simulink model "Charge_2_V1"  (R2017b)
settings: Solver=FixedStepDiscrete  StartTime=0.0  StopTime=1  FixedStep=0.001  RelTol=1e-3
PreLoadFcn:
  | librarySetup
  | eval([bdroot,'_startup']) %Calling [modelName]_startup.m
undefined symbols (not defined in the file or in its folder): A0, A1, Car1__Authorize, Car2_Authorize, CON2, CON3, CON4, Control_Mode_In, CurrentSP, D10, D12, D13, D2, D3, D4, D5, D6, D7, D8, Frequency_High_Point, Frequency_Low_Point, Frequency_Mid_high, Frequency_Mid_low, HVol_High_Point, HVol_Low_Point, HVol_Mid_high, HVol_Mid_low, HVoltage_Factor, SeconCar_ThreePhase, V_Current_five, V_Current_four, V_Current_one, V_Current_six, V_Current_three, V_Current_two, V_Frequency, V_MaxPliot, V_MinPliot, Vol_High_Point, Vol_Low_Point, Vol_Mid_high, Vol_Mid_low, Voltage_Factor, Voltage_Mode_Test
libraries: simulink x331, HANcoder_STM32_Target x30, powerlib_meascontrol x8, simulink_extras x2
(part 5 of 13)

== system Charge_2_V1/HANcoder STM32 Target - E407-STM32 algorithm/Energy Meter1/Energy_Meter_Recieve/Current_Meter/Read_Gyro13 ==
  Trigger : TriggerPort  VariantControl=Variant
  UART receive : Subsystem  AncestorBlock=HANcoder_STM32_Target/STM32-E407/UART/UART receive  mask(UART receive){channel=UART2: Con. PD-8 & Con. PD-9 (PD5 & PD6), useStatusOut=off, tsamp=-1}
      mask prompts: useStatusOut "Use status outport"; tsamp "Sample time"
      mask help:
      | Function
      | ==========
      | Reads a byte from the UART reception buffer.
      |
      | Parameters per channel
      | ======================
      | - Select channel
      | - Select if the status output should be enabled.
      |
      | Outputs
      | =======
      | - The value of the receive byte.
      | - When the status output is 0, the reception buffer was empty.
      mask init:
      | uartChannelInfoStr = sfcn_uart_receive_mcb(2, channel, useStatusOut);
      settings: MoveFcn=drawLogos
      mask Help: web('sfcn_uart_receive.html')
      mask TypeOptions channel: UART1: Con. 3-D1 & Con. 3-D0 (PB6 & PB7) | UART2: Con. PD-8 & Con. PD-9 (PD5 & PD6) | UART3: Con. PD-11 & Con. PD-12 (PD8 & PD9) | UART6: Con. UEXT-3 & Con. UEXT-4 (PC6 & PC7)
      mask Display: fprintf('UART receive\n%s', uartChannelInfoStr);patch([240 246 246],[8 14 2],[1 0 0]);patch([248 248 254],[14 2 8],[0 0 0.35]);
  Out1 : Outport
  wires:
  UART receive/1(Out1) -> Out1/1

== system Charge_2_V1/HANcoder STM32 Target - E407-STM32 algorithm/Energy Meter1/Energy_Meter_Recieve/Current_Meter/Read_Gyro14 ==
  Trigger : TriggerPort  VariantControl=Variant
  UART receive : Subsystem  AncestorBlock=HANcoder_STM32_Target/STM32-E407/UART/UART receive  mask(UART receive){channel=UART2: Con. PD-8 & Con. PD-9 (PD5 & PD6), useStatusOut=off, tsamp=-1}
      mask prompts: useStatusOut "Use status outport"; tsamp "Sample time"
      mask help:
      | Function
      | ==========
      | Reads a byte from the UART reception buffer.
      |
      | Parameters per channel
      | ======================
      | - Select channel
      | - Select if the status output should be enabled.
      |
      | Outputs
      | =======
      | - The value of the receive byte.
      | - When the status output is 0, the reception buffer was empty.
      mask init:
      | uartChannelInfoStr = sfcn_uart_receive_mcb(2, channel, useStatusOut);
      settings: MoveFcn=drawLogos
      mask Help: web('sfcn_uart_receive.html')
      mask TypeOptions channel: UART1: Con. 3-D1 & Con. 3-D0 (PB6 & PB7) | UART2: Con. PD-8 & Con. PD-9 (PD5 & PD6) | UART3: Con. PD-11 & Con. PD-12 (PD8 & PD9) | UART6: Con. UEXT-3 & Con. UEXT-4 (PC6 & PC7)
      mask Display: fprintf('UART receive\n%s', uartChannelInfoStr);patch([240 246 246],[8 14 2],[1 0 0]);patch([248 248 254],[14 2 8],[0 0 0.35]);
  Out1 : Outport
  wires:
  UART receive/1(Out1) -> Out1/1

== system Charge_2_V1/HANcoder STM32 Target - E407-STM32 algorithm/Energy Meter1/Energy_Meter_Recieve/Current_Meter/Read_Gyro15 ==
  Trigger : TriggerPort  VariantControl=Variant
  UART receive : Subsystem  AncestorBlock=HANcoder_STM32_Target/STM32-E407/UART/UART receive  mask(UART receive){channel=UART2: Con. PD-8 & Con. PD-9 (PD5 & PD6), useStatusOut=off, tsamp=-1}
      mask prompts: useStatusOut "Use status outport"; tsamp "Sample time"
      mask help:
      | Function
      | ==========
      | Reads a byte from the UART reception buffer.
      |
      | Parameters per channel
      | ======================
      | - Select channel
      | - Select if the status output should be enabled.
      |
      | Outputs
      | =======
      | - The value of the receive byte.
      | - When the status output is 0, the reception buffer was empty.
      mask init:
      | uartChannelInfoStr = sfcn_uart_receive_mcb(2, channel, useStatusOut);
      settings: MoveFcn=drawLogos
      mask Help: web('sfcn_uart_receive.html')
      mask TypeOptions channel: UART1: Con. 3-D1 & Con. 3-D0 (PB6 & PB7) | UART2: Con. PD-8 & Con. PD-9 (PD5 & PD6) | UART3: Con. PD-11 & Con. PD-12 (PD8 & PD9) | UART6: Con. UEXT-3 & Con. UEXT-4 (PC6 & PC7)
      mask Display: fprintf('UART receive\n%s', uartChannelInfoStr);patch([240 246 246],[8 14 2],[1 0 0]);patch([248 248 254],[14 2 8],[0 0 0.35]);
  Out1 : Outport
  wires:
  UART receive/1(Out1) -> Out1/1

== system Charge_2_V1/HANcoder STM32 Target - E407-STM32 algorithm/Energy Meter1/Energy_Meter_Recieve/Current_Meter/Read_Gyro16 ==
  Trigger : TriggerPort  VariantControl=Variant
  UART receive : Subsystem  AncestorBlock=HANcoder_STM32_Target/STM32-E407/UART/UART receive  mask(UART receive){channel=UART2: Con. PD-8 & Con. PD-9 (PD5 & PD6), useStatusOut=off, tsamp=-1}
      mask prompts: useStatusOut "Use status outport"; tsamp "Sample time"
      mask help:
      | Function
      | ==========
      | Reads a byte from the UART reception buffer.
      |
      | Parameters per channel
      | ======================
      | - Select channel
      | - Select if the status output should be enabled.
      |
      | Outputs
      | =======
      | - The value of the receive byte.
      | - When the status output is 0, the reception buffer was empty.
      mask init:
      | uartChannelInfoStr = sfcn_uart_receive_mcb(2, channel, useStatusOut);
      settings: MoveFcn=drawLogos
      mask Help: web('sfcn_uart_receive.html')
      mask TypeOptions channel: UART1: Con. 3-D1 & Con. 3-D0 (PB6 & PB7) | UART2: Con. PD-8 & Con. PD-9 (PD5 & PD6) | UART3: Con. PD-11 & Con. PD-12 (PD8 & PD9) | UART6: Con. UEXT-3 & Con. UEXT-4 (PC6 & PC7)
      mask Display: fprintf('UART receive\n%s', uartChannelInfoStr);patch([240 246 246],[8 14 2],[1 0 0]);patch([248 248 254],[14 2 8],[0 0 0.35]);
  Out1 : Outport
  wires:
  UART receive/1(Out1) -> Out1/1

== system Charge_2_V1/HANcoder STM32 Target - E407-STM32 algorithm/Energy Meter1/Energy_Meter_Recieve/Current_Meter/Read_Gyro17 ==
  Trigger : TriggerPort  VariantControl=Variant
  UART receive : Subsystem  AncestorBlock=HANcoder_STM32_Target/STM32-E407/UART/UART receive  mask(UART receive){channel=UART2: Con. PD-8 & Con. PD-9 (PD5 & PD6), useStatusOut=off, tsamp=-1}
      mask prompts: useStatusOut "Use status outport"; tsamp "Sample time"
      mask help:
      | Function
      | ==========
      | Reads a byte from the UART reception buffer.
      |
      | Parameters per channel
      | ======================
      | - Select channel
      | - Select if the status output should be enabled.
      |
      | Outputs
      | =======
      | - The value of the receive byte.
      | - When the status output is 0, the reception buffer was empty.
      mask init:
      | uartChannelInfoStr = sfcn_uart_receive_mcb(2, channel, useStatusOut);
      settings: MoveFcn=drawLogos
      mask Help: web('sfcn_uart_receive.html')
      mask TypeOptions channel: UART1: Con. 3-D1 & Con. 3-D0 (PB6 & PB7) | UART2: Con. PD-8 & Con. PD-9 (PD5 & PD6) | UART3: Con. PD-11 & Con. PD-12 (PD8 & PD9) | UART6: Con. UEXT-3 & Con. UEXT-4 (PC6 & PC7)
      mask Display: fprintf('UART receive\n%s', uartChannelInfoStr);patch([240 246 246],[8 14 2],[1 0 0]);patch([248 248 254],[14 2 8],[0 0 0.35]);
  Out1 : Outport
  wires:
  UART receive/1(Out1) -> Out1/1

== system Charge_2_V1/HANcoder STM32 Target - E407-STM32 algorithm/Energy Meter1/Energy_Meter_Recieve/Current_Meter/Read_Gyro18 ==
  Trigger : TriggerPort  VariantControl=Variant
  UART receive : Subsystem  AncestorBlock=HANcoder_STM32_Target/STM32-E407/UART/UART receive  mask(UART receive){channel=UART2: Con. PD-8 & Con. PD-9 (PD5 & PD6), useStatusOut=off, tsamp=-1}
      mask prompts: useStatusOut "Use status outport"; tsamp "Sample time"
      mask help:
      | Function
      | ==========
      | Reads a byte from the UART reception buffer.
      |
      | Parameters per channel
      | ======================
      | - Select channel
      | - Select if the status output should be enabled.
      |
      | Outputs
      | =======
      | - The value of the receive byte.
      | - When the status output is 0, the reception buffer was empty.
      mask init:
      | uartChannelInfoStr = sfcn_uart_receive_mcb(2, channel, useStatusOut);
      settings: MoveFcn=drawLogos
      mask Help: web('sfcn_uart_receive.html')
      mask TypeOptions channel: UART1: Con. 3-D1 & Con. 3-D0 (PB6 & PB7) | UART2: Con. PD-8 & Con. PD-9 (PD5 & PD6) | UART3: Con. PD-11 & Con. PD-12 (PD8 & PD9) | UART6: Con. UEXT-3 & Con. UEXT-4 (PC6 & PC7)
      mask Display: fprintf('UART receive\n%s', uartChannelInfoStr);patch([240 246 246],[8 14 2],[1 0 0]);patch([248 248 254],[14 2 8],[0 0 0.35]);
  Out1 : Outport
  wires:
  UART receive/1(Out1) -> Out1/1

== system Charge_2_V1/HANcoder STM32 Target - E407-STM32 algorithm/Energy Meter1/Energy_Meter_Recieve/Current_Meter/Read_Gyro2 ==
  Trigger : TriggerPort  VariantControl=Variant
  UART receive : Subsystem  AncestorBlock=HANcoder_STM32_Target/STM32-E407/UART/UART receive  mask(UART receive){channel=UART2: Con. PD-8 & Con. PD-9 (PD5 & PD6), useStatusOut=off, tsamp=-1}
      mask prompts: useStatusOut "Use status outport"; tsamp "Sample time"
      mask help:
      | Function
      | ==========
      | Reads a byte from the UART reception buffer.
      |
      | Parameters per channel
      | ======================
      | - Select channel
      | - Select if the status output should be enabled.
      |
      | Outputs
      | =======
      | - The value of the receive byte.
      | - When the status output is 0, the reception buffer was empty.
      mask init:
      | uartChannelInfoStr = sfcn_uart_receive_mcb(2, channel, useStatusOut);
      settings: MoveFcn=drawLogos
      mask Help: web('sfcn_uart_receive.html')
      mask TypeOptions channel: UART1: Con. 3-D1 & Con. 3-D0 (PB6 & PB7) | UART2: Con. PD-8 & Con. PD-9 (PD5 & PD6) | UART3: Con. PD-11 & Con. PD-12 (PD8 & PD9) | UART6: Con. UEXT-3 & Con. UEXT-4 (PC6 & PC7)
      mask Display: fprintf('UART receive\n%s', uartChannelInfoStr);patch([240 246 246],[8 14 2],[1 0 0]);patch([248 248 254],[14 2 8],[0 0 0.35]);
  Out1 : Outport
  wires:
  UART receive/1(Out1) -> Out1/1

== system Charge_2_V1/HANcoder STM32 Target - E407-STM32 algorithm/Energy Meter1/Energy_Meter_Recieve/Current_Meter/Read_Gyro3 ==
  Trigger : TriggerPort  VariantControl=Variant
  UART receive : Subsystem  AncestorBlock=HANcoder_STM32_Target/STM32-E407/UART/UART receive  mask(UART receive){channel=UART2: Con. PD-8 & Con. PD-9 (PD5 & PD6), useStatusOut=off, tsamp=-1}
      mask prompts: useStatusOut "Use status outport"; tsamp "Sample time"
      mask help:
      | Function
      | ==========
      | Reads a byte from the UART reception buffer.
      |
      | Parameters per channel
      | ======================
      | - Select channel
      | - Select if the status output should be enabled.
      |
      | Outputs
      | =======
      | - The value of the receive byte.
      | - When the status output is 0, the reception buffer was empty.
      mask init:
      | uartChannelInfoStr = sfcn_uart_receive_mcb(2, channel, useStatusOut);
      settings: MoveFcn=drawLogos
      mask Help: web('sfcn_uart_receive.html')
      mask TypeOptions channel: UART1: Con. 3-D1 & Con. 3-D0 (PB6 & PB7) | UART2: Con. PD-8 & Con. PD-9 (PD5 & PD6) | UART3: Con. PD-11 & Con. PD-12 (PD8 & PD9) | UART6: Con. UEXT-3 & Con. UEXT-4 (PC6 & PC7)
      mask Display: fprintf('UART receive\n%s', uartChannelInfoStr);patch([240 246 246],[8 14 2],[1 0 0]);patch([248 248 254],[14 2 8],[0 0 0.35]);
  Out1 : Outport
  wires:
  UART receive/1(Out1) -> Out1/1

== system Charge_2_V1/HANcoder STM32 Target - E407-STM32 algorithm/Energy Meter1/Energy_Meter_Recieve/Current_Meter/Read_Gyro4 ==
  Trigger : TriggerPort  VariantControl=Variant
  UART receive : Subsystem  AncestorBlock=HANcoder_STM32_Target/STM32-E407/UART/UART receive  mask(UART receive){channel=UART2: Con. PD-8 & Con. PD-9 (PD5 & PD6), useStatusOut=off, tsamp=-1}
      mask prompts: useStatusOut "Use status outport"; tsamp "Sample time"
      mask help:
      | Function
      | ==========
      | Reads a byte from the UART reception buffer.
      |
      | Parameters per channel
      | ======================
      | - Select channel
      | - Select if the status output should be enabled.
      |
      | Outputs
      | =======
      | - The value of the receive byte.
      | - When the status output is 0, the reception buffer was empty.
      mask init:
      | uartChannelInfoStr = sfcn_uart_receive_mcb(2, channel, useStatusOut);
      settings: MoveFcn=drawLogos
      mask Help: web('sfcn_uart_receive.html')
      mask TypeOptions channel: UART1: Con. 3-D1 & Con. 3-D0 (PB6 & PB7) | UART2: Con. PD-8 & Con. PD-9 (PD5 & PD6) | UART3: Con. PD-11 & Con. PD-12 (PD8 & PD9) | UART6: Con. UEXT-3 & Con. UEXT-4 (PC6 & PC7)
      mask Display: fprintf('UART receive\n%s', uartChannelInfoStr);patch([240 246 246],[8 14 2],[1 0 0]);patch([248 248 254],[14 2 8],[0 0 0.35]);
  Out1 : Outport
  wires:
  UART receive/1(Out1) -> Out1/1

== system Charge_2_V1/HANcoder STM32 Target - E407-STM32 algorithm/Energy Meter1/Energy_Meter_Recieve/Current_Meter/Read_Gyro5 ==
  Trigger : TriggerPort  VariantControl=Variant
  UART receive : Subsystem  AncestorBlock=HANcoder_STM32_Target/STM32-E407/UART/UART receive  mask(UART receive){channel=UART2: Con. PD-8 & Con. PD-9 (PD5 & PD6), useStatusOut=off, tsamp=-1}
      mask prompts: useStatusOut "Use status outport"; tsamp "Sample time"
      mask help:
      | Function
      | ==========
      | Reads a byte from the UART reception buffer.
      |
      | Parameters per channel
      | ======================
      | - Select channel
      | - Select if the status output should be enabled.
      |
      | Outputs
      | =======
      | - The value of the receive byte.
      | - When the status output is 0, the reception buffer was empty.
      mask init:
      | uartChannelInfoStr = sfcn_uart_receive_mcb(2, channel, useStatusOut);
      settings: MoveFcn=drawLogos
      mask Help: web('sfcn_uart_receive.html')
      mask TypeOptions channel: UART1: Con. 3-D1 & Con. 3-D0 (PB6 & PB7) | UART2: Con. PD-8 & Con. PD-9 (PD5 & PD6) | UART3: Con. PD-11 & Con. PD-12 (PD8 & PD9) | UART6: Con. UEXT-3 & Con. UEXT-4 (PC6 & PC7)
      mask Display: fprintf('UART receive\n%s', uartChannelInfoStr);patch([240 246 246],[8 14 2],[1 0 0]);patch([248 248 254],[14 2 8],[0 0 0.35]);
  Out1 : Outport
  wires:
  UART receive/1(Out1) -> Out1/1

== system Charge_2_V1/HANcoder STM32 Target - E407-STM32 algorithm/Energy Meter1/Energy_Meter_Recieve/Current_Meter/Read_Gyro6 ==
  Trigger : TriggerPort  VariantControl=Variant
  UART receive : Subsystem  AncestorBlock=HANcoder_STM32_Target/STM32-E407/UART/UART receive  mask(UART receive){channel=UART2: Con. PD-8 & Con. PD-9 (PD5 & PD6), useStatusOut=off, tsamp=-1}
      mask prompts: useStatusOut "Use status outport"; tsamp "Sample time"
      mask help:
      | Function
      | ==========
      | Reads a byte from the UART reception buffer.
      |
      | Parameters per channel
      | ======================
      | - Select channel
      | - Select if the status output should be enabled.
      |
      | Outputs
      | =======
      | - The value of the receive byte.
      | - When the status output is 0, the reception buffer was empty.
      mask init:
      | uartChannelInfoStr = sfcn_uart_receive_mcb(2, channel, useStatusOut);
      settings: MoveFcn=drawLogos
      mask Help: web('sfcn_uart_receive.html')
      mask TypeOptions channel: UART1: Con. 3-D1 & Con. 3-D0 (PB6 & PB7) | UART2: Con. PD-8 & Con. PD-9 (PD5 & PD6) | UART3: Con. PD-11 & Con. PD-12 (PD8 & PD9) | UART6: Con. UEXT-3 & Con. UEXT-4 (PC6 & PC7)
      mask Display: fprintf('UART receive\n%s', uartChannelInfoStr);patch([240 246 246],[8 14 2],[1 0 0]);patch([248 248 254],[14 2 8],[0 0 0.35]);
  Out1 : Outport
  wires:
  UART receive/1(Out1) -> Out1/1

== system Charge_2_V1/HANcoder STM32 Target - E407-STM32 algorithm/Energy Meter1/Energy_Meter_Recieve/Current_Meter/Read_Gyro7 ==
  Trigger : TriggerPort  VariantControl=Variant
  UART receive : Subsystem  AncestorBlock=HANcoder_STM32_Target/STM32-E407/UART/UART receive  mask(UART receive){channel=UART2: Con. PD-8 & Con. PD-9 (PD5 & PD6), useStatusOut=off, tsamp=-1}
      mask prompts: useStatusOut "Use status outport"; tsamp "Sample time"
      mask help:
      | Function
      | ==========
      | Reads a byte from the UART reception buffer.
      |
      | Parameters per channel
      | ======================
      | - Select channel
      | - Select if the status output should be enabled.
      |
      | Outputs
      | =======
      | - The value of the receive byte.
      | - When the status output is 0, the reception buffer was empty.
      mask init:
      | uartChannelInfoStr = sfcn_uart_receive_mcb(2, channel, useStatusOut);
      settings: MoveFcn=drawLogos
      mask Help: web('sfcn_uart_receive.html')
      mask TypeOptions channel: UART1: Con. 3-D1 & Con. 3-D0 (PB6 & PB7) | UART2: Con. PD-8 & Con. PD-9 (PD5 & PD6) | UART3: Con. PD-11 & Con. PD-12 (PD8 & PD9) | UART6: Con. UEXT-3 & Con. UEXT-4 (PC6 & PC7)
      mask Display: fprintf('UART receive\n%s', uartChannelInfoStr);patch([240 246 246],[8 14 2],[1 0 0]);patch([248 248 254],[14 2 8],[0 0 0.35]);
  Out1 : Outport
  wires:
  UART receive/1(Out1) -> Out1/1

== system Charge_2_V1/HANcoder STM32 Target - E407-STM32 algorithm/Energy Meter1/Energy_Meter_Recieve/Current_Meter/Read_Gyro8 ==
  Trigger : TriggerPort  VariantControl=Variant
  UART receive : Subsystem  AncestorBlock=HANcoder_STM32_Target/STM32-E407/UART/UART receive  mask(UART receive){channel=UART2: Con. PD-8 & Con. PD-9 (PD5 & PD6), useStatusOut=off, tsamp=-1}
      mask prompts: useStatusOut "Use status outport"; tsamp "Sample time"
      mask help:
      | Function
      | ==========
      | Reads a byte from the UART reception buffer.
      |
      | Parameters per channel
      | ======================
      | - Select channel
      | - Select if the status output should be enabled.
      |
      | Outputs
      | =======
      | - The value of the receive byte.
      | - When the status output is 0, the reception buffer was empty.
      mask init:
      | uartChannelInfoStr = sfcn_uart_receive_mcb(2, channel, useStatusOut);
      settings: MoveFcn=drawLogos
      mask Help: web('sfcn_uart_receive.html')
      mask TypeOptions channel: UART1: Con. 3-D1 & Con. 3-D0 (PB6 & PB7) | UART2: Con. PD-8 & Con. PD-9 (PD5 & PD6) | UART3: Con. PD-11 & Con. PD-12 (PD8 & PD9) | UART6: Con. UEXT-3 & Con. UEXT-4 (PC6 & PC7)
      mask Display: fprintf('UART receive\n%s', uartChannelInfoStr);patch([240 246 246],[8 14 2],[1 0 0]);patch([248 248 254],[14 2 8],[0 0 0.35]);
  Out1 : Outport
  wires:
  UART receive/1(Out1) -> Out1/1

== system Charge_2_V1/HANcoder STM32 Target - E407-STM32 algorithm/Energy Meter1/Energy_Meter_Recieve/Current_Meter/Read_Gyro9 ==
  Trigger : TriggerPort  VariantControl=Variant
  UART receive : Subsystem  AncestorBlock=HANcoder_STM32_Target/STM32-E407/UART/UART receive  mask(UART receive){channel=UART2: Con. PD-8 & Con. PD-9 (PD5 & PD6), useStatusOut=off, tsamp=-1}
      mask prompts: useStatusOut "Use status outport"; tsamp "Sample time"
      mask help:
      | Function
      | ==========
      | Reads a byte from the UART reception buffer.
      |
      | Parameters per channel
      | ======================
      | - Select channel
      | - Select if the status output should be enabled.
      |
      | Outputs
      | =======
      | - The value of the receive byte.
      | - When the status output is 0, the reception buffer was empty.
      mask init:
      | uartChannelInfoStr = sfcn_uart_receive_mcb(2, channel, useStatusOut);
      settings: MoveFcn=drawLogos
      mask Help: web('sfcn_uart_receive.html')
      mask TypeOptions channel: UART1: Con. 3-D1 & Con. 3-D0 (PB6 & PB7) | UART2: Con. PD-8 & Con. PD-9 (PD5 & PD6) | UART3: Con. PD-11 & Con. PD-12 (PD8 & PD9) | UART6: Con. UEXT-3 & Con. UEXT-4 (PC6 & PC7)
      mask Display: fprintf('UART receive\n%s', uartChannelInfoStr);patch([240 246 246],[8 14 2],[1 0 0]);patch([248 248 254],[14 2 8],[0 0 0.35]);
  Out1 : Outport
  wires:
  UART receive/1(Out1) -> Out1/1

== system Charge_2_V1/HANcoder STM32 Target - E407-STM32 algorithm/Energy Meter1/Energy_Meter_Recieve/Fequency/Read_Gyro ==
  Trigger : TriggerPort  VariantControl=Variant
  UART receive : Subsystem  AncestorBlock=HANcoder_STM32_Target/STM32-E407/UART/UART receive  mask(UART receive){channel=UART2: Con. PD-8 & Con. PD-9 (PD5 & PD6), useStatusOut=off, tsamp=-1}
      mask prompts: useStatusOut "Use status outport"; tsamp "Sample time"
      mask help:
      | Function
      | ==========
      | Reads a byte from the UART reception buffer.
      |
      | Parameters per channel
      | ======================
      | - Select channel
      | - Select if the status output should be enabled.
      |
      | Outputs
      | =======
      | - The value of the receive byte.
      | - When the status output is 0, the reception buffer was empty.
      mask init:
      | uartChannelInfoStr = sfcn_uart_receive_mcb(2, channel, useStatusOut);
      settings: MoveFcn=drawLogos
      mask Help: web('sfcn_uart_receive.html')
      mask TypeOptions channel: UART1: Con. 3-D1 & Con. 3-D0 (PB6 & PB7) | UART2: Con. PD-8 & Con. PD-9 (PD5 & PD6) | UART3: Con. PD-11 & Con. PD-12 (PD8 & PD9) | UART6: Con. UEXT-3 & Con. UEXT-4 (PC6 & PC7)
      mask Display: fprintf('UART receive\n%s', uartChannelInfoStr);patch([240 246 246],[8 14 2],[1 0 0]);patch([248 248 254],[14 2 8],[0 0 0.35]);
  Out1 : Outport
  wires:
  UART receive/1(Out1) -> Out1/1

== system Charge_2_V1/HANcoder STM32 Target - E407-STM32 algorithm/Energy Meter1/Energy_Meter_Recieve/Fequency/Read_Gyro1 ==
  Trigger : TriggerPort  VariantControl=Variant
  UART receive : Subsystem  AncestorBlock=HANcoder_STM32_Target/STM32-E407/UART/UART receive  mask(UART receive){channel=UART2: Con. PD-8 & Con. PD-9 (PD5 & PD6), useStatusOut=off, tsamp=-1}
      mask prompts: useStatusOut "Use status outport"; tsamp "Sample time"
      mask help:
      | Function
      | ==========
      | Reads a byte from the UART reception buffer.
      |
      | Parameters per channel
      | ======================
      | - Select channel
      | - Select if the status output should be enabled.
      |
      | Outputs
      | =======
      | - The value of the receive byte.
      | - When the status output is 0, the reception buffer was empty.
      mask init:
      | uartChannelInfoStr = sfcn_uart_receive_mcb(2, channel, useStatusOut);
      settings: MoveFcn=drawLogos
      mask Help: web('sfcn_uart_receive.html')
      mask TypeOptions channel: UART1: Con. 3-D1 & Con. 3-D0 (PB6 & PB7) | UART2: Con. PD-8 & Con. PD-9 (PD5 & PD6) | UART3: Con. PD-11 & Con. PD-12 (PD8 & PD9) | UART6: Con. UEXT-3 & Con. UEXT-4 (PC6 & PC7)
      mask Display: fprintf('UART receive\n%s', uartChannelInfoStr);patch([240 246 246],[8 14 2],[1 0 0]);patch([248 248 254],[14 2 8],[0 0 0.35]);
  Out1 : Outport
  wires:
  UART receive/1(Out1) -> Out1/1

== system Charge_2_V1/HANcoder STM32 Target - E407-STM32 algorithm/Energy Meter1/Energy_Meter_Recieve/Fequency/Read_Gyro10 ==
  Trigger : TriggerPort  VariantControl=Variant
  UART receive : Subsystem  AncestorBlock=HANcoder_STM32_Target/STM32-E407/UART/UART receive  mask(UART receive){channel=UART2: Con. PD-8 & Con. PD-9 (PD5 & PD6), useStatusOut=off, tsamp=-1}
      mask prompts: useStatusOut "Use status outport"; tsamp "Sample time"
      mask help:
      | Function
      | ==========
      | Reads a byte from the UART reception buffer.
      |
      | Parameters per channel
      | ======================
      | - Select channel
      | - Select if the status output should be enabled.
      |
      | Outputs
      | =======
      | - The value of the receive byte.
      | - When the status output is 0, the reception buffer was empty.
      mask init:
      | uartChannelInfoStr = sfcn_uart_receive_mcb(2, channel, useStatusOut);
      settings: MoveFcn=drawLogos
      mask Help: web('sfcn_uart_receive.html')
      mask TypeOptions channel: UART1: Con. 3-D1 & Con. 3-D0 (PB6 & PB7) | UART2: Con. PD-8 & Con. PD-9 (PD5 & PD6) | UART3: Con. PD-11 & Con. PD-12 (PD8 & PD9) | UART6: Con. UEXT-3 & Con. UEXT-4 (PC6 & PC7)
      mask Display: fprintf('UART receive\n%s', uartChannelInfoStr);patch([240 246 246],[8 14 2],[1 0 0]);patch([248 248 254],[14 2 8],[0 0 0.35]);
  Out1 : Outport
  wires:
  UART receive/1(Out1) -> Out1/1

== system Charge_2_V1/HANcoder STM32 Target - E407-STM32 algorithm/Energy Meter1/Energy_Meter_Recieve/Fequency/Read_Gyro2 ==
  Trigger : TriggerPort  VariantControl=Variant
  UART receive : Subsystem  AncestorBlock=HANcoder_STM32_Target/STM32-E407/UART/UART receive  mask(UART receive){channel=UART2: Con. PD-8 & Con. PD-9 (PD5 & PD6), useStatusOut=off, tsamp=-1}
      mask prompts: useStatusOut "Use status outport"; tsamp "Sample time"
      mask help:
      | Function
      | ==========
      | Reads a byte from the UART reception buffer.
      |
      | Parameters per channel
      | ======================
      | - Select channel
      | - Select if the status output should be enabled.
      |
      | Outputs
      | =======
      | - The value of the receive byte.
      | - When the status output is 0, the reception buffer was empty.
      mask init:
      | uartChannelInfoStr = sfcn_uart_receive_mcb(2, channel, useStatusOut);
      settings: MoveFcn=drawLogos
      mask Help: web('sfcn_uart_receive.html')
      mask TypeOptions channel: UART1: Con. 3-D1 & Con. 3-D0 (PB6 & PB7) | UART2: Con. PD-8 & Con. PD-9 (PD5 & PD6) | UART3: Con. PD-11 & Con. PD-12 (PD8 & PD9) | UART6: Con. UEXT-3 & Con. UEXT-4 (PC6 & PC7)
      mask Display: fprintf('UART receive\n%s', uartChannelInfoStr);patch([240 246 246],[8 14 2],[1 0 0]);patch([248 248 254],[14 2 8],[0 0 0.35]);
  Out1 : Outport
  wires:
  UART receive/1(Out1) -> Out1/1

== system Charge_2_V1/HANcoder STM32 Target - E407-STM32 algorithm/Energy Meter1/Energy_Meter_Recieve/Fequency/Read_Gyro3 ==
  Trigger : TriggerPort  VariantControl=Variant
  UART receive : Subsystem  AncestorBlock=HANcoder_STM32_Target/STM32-E407/UART/UART receive  mask(UART receive){channel=UART2: Con. PD-8 & Con. PD-9 (PD5 & PD6), useStatusOut=off, tsamp=-1}
      mask prompts: useStatusOut "Use status outport"; tsamp "Sample time"
      mask help:
      | Function
      | ==========
      | Reads a byte from the UART reception buffer.
      |
      | Parameters per channel
      | ======================
      | - Select channel
      | - Select if the status output should be enabled.
      |
      | Outputs
      | =======
      | - The value of the receive byte.
      | - When the status output is 0, the reception buffer was empty.
      mask init:
      | uartChannelInfoStr = sfcn_uart_receive_mcb(2, channel, useStatusOut);
      settings: MoveFcn=drawLogos
      mask Help: web('sfcn_uart_receive.html')
      mask TypeOptions channel: UART1: Con. 3-D1 & Con. 3-D0 (PB6 & PB7) | UART2: Con. PD-8 & Con. PD-9 (PD5 & PD6) | UART3: Con. PD-11 & Con. PD-12 (PD8 & PD9) | UART6: Con. UEXT-3 & Con. UEXT-4 (PC6 & PC7)
      mask Display: fprintf('UART receive\n%s', uartChannelInfoStr);patch([240 246 246],[8 14 2],[1 0 0]);patch([248 248 254],[14 2 8],[0 0 0.35]);
  Out1 : Outport
  wires:
  UART receive/1(Out1) -> Out1/1

== system Charge_2_V1/HANcoder STM32 Target - E407-STM32 algorithm/Energy Meter1/Energy_Meter_Recieve/Fequency/Read_Gyro4 ==
  Trigger : TriggerPort  VariantControl=Variant
  UART receive : Subsystem  AncestorBlock=HANcoder_STM32_Target/STM32-E407/UART/UART receive  mask(UART receive){channel=UART2: Con. PD-8 & Con. PD-9 (PD5 & PD6), useStatusOut=off, tsamp=-1}
      mask prompts: useStatusOut "Use status outport"; tsamp "Sample time"
      mask help:
      | Function
      | ==========
      | Reads a byte from the UART reception buffer.
      |
      | Parameters per channel
      | ======================
      | - Select channel
      | - Select if the status output should be enabled.
      |
      | Outputs
      | =======
      | - The value of the receive byte.
      | - When the status output is 0, the reception buffer was empty.
      mask init:
      | uartChannelInfoStr = sfcn_uart_receive_mcb(2, channel, useStatusOut);
      settings: MoveFcn=drawLogos
      mask Help: web('sfcn_uart_receive.html')
      mask TypeOptions channel: UART1: Con. 3-D1 & Con. 3-D0 (PB6 & PB7) | UART2: Con. PD-8 & Con. PD-9 (PD5 & PD6) | UART3: Con. PD-11 & Con. PD-12 (PD8 & PD9) | UART6: Con. UEXT-3 & Con. UEXT-4 (PC6 & PC7)
      mask Display: fprintf('UART receive\n%s', uartChannelInfoStr);patch([240 246 246],[8 14 2],[1 0 0]);patch([248 248 254],[14 2 8],[0 0 0.35]);
  Out1 : Outport
  wires:
  UART receive/1(Out1) -> Out1/1

== system Charge_2_V1/HANcoder STM32 Target - E407-STM32 algorithm/Energy Meter1/Energy_Meter_Recieve/Fequency/Read_Gyro5 ==
  Trigger : TriggerPort  VariantControl=Variant
  UART receive : Subsystem  AncestorBlock=HANcoder_STM32_Target/STM32-E407/UART/UART receive  mask(UART receive){channel=UART2: Con. PD-8 & Con. PD-9 (PD5 & PD6), useStatusOut=off, tsamp=-1}
      mask prompts: useStatusOut "Use status outport"; tsamp "Sample time"
      mask help:
      | Function
      | ==========
      | Reads a byte from the UART reception buffer.
      |
      | Parameters per channel
      | ======================
      | - Select channel
      | - Select if the status output should be enabled.
      |
      | Outputs
      | =======
      | - The value of the receive byte.
      | - When the status output is 0, the reception buffer was empty.
      mask init:
      | uartChannelInfoStr = sfcn_uart_receive_mcb(2, channel, useStatusOut);
      settings: MoveFcn=drawLogos
      mask Help: web('sfcn_uart_receive.html')
      mask TypeOptions channel: UART1: Con. 3-D1 & Con. 3-D0 (PB6 & PB7) | UART2: Con. PD-8 & Con. PD-9 (PD5 & PD6) | UART3: Con. PD-11 & Con. PD-12 (PD8 & PD9) | UART6: Con. UEXT-3 & Con. UEXT-4 (PC6 & PC7)
      mask Display: fprintf('UART receive\n%s', uartChannelInfoStr);patch([240 246 246],[8 14 2],[1 0 0]);patch([248 248 254],[14 2 8],[0 0 0.35]);
  Out1 : Outport
  wires:
  UART receive/1(Out1) -> Out1/1

== system Charge_2_V1/HANcoder STM32 Target - E407-STM32 algorithm/Energy Meter1/Energy_Meter_Recieve/Fequency/Read_Gyro6 ==
  Trigger : TriggerPort  VariantControl=Variant
  UART receive : Subsystem  AncestorBlock=HANcoder_STM32_Target/STM32-E407/UART/UART receive  mask(UART receive){channel=UART2: Con. PD-8 & Con. PD-9 (PD5 & PD6), useStatusOut=off, tsamp=-1}
      mask prompts: useStatusOut "Use status outport"; tsamp "Sample time"
      mask help:
      | Function
      | ==========
      | Reads a byte from the UART reception buffer.
      |
      | Parameters per channel
      | ======================
      | - Select channel
      | - Select if the status output should be enabled.
      |
      | Outputs
      | =======
      | - The value of the receive byte.
      | - When the status output is 0, the reception buffer was empty.
      mask init:
      | uartChannelInfoStr = sfcn_uart_receive_mcb(2, channel, useStatusOut);
      settings: MoveFcn=drawLogos
      mask Help: web('sfcn_uart_receive.html')
      mask TypeOptions channel: UART1: Con. 3-D1 & Con. 3-D0 (PB6 & PB7) | UART2: Con. PD-8 & Con. PD-9 (PD5 & PD6) | UART3: Con. PD-11 & Con. PD-12 (PD8 & PD9) | UART6: Con. UEXT-3 & Con. UEXT-4 (PC6 & PC7)
      mask Display: fprintf('UART receive\n%s', uartChannelInfoStr);patch([240 246 246],[8 14 2],[1 0 0]);patch([248 248 254],[14 2 8],[0 0 0.35]);
  Out1 : Outport
  wires:
  UART receive/1(Out1) -> Out1/1

== system Charge_2_V1/HANcoder STM32 Target - E407-STM32 algorithm/Energy Meter1/Energy_Meter_Recieve/Fequency/Read_Gyro7 ==
  Trigger : TriggerPort  VariantControl=Variant
  UART receive : Subsystem  AncestorBlock=HANcoder_STM32_Target/STM32-E407/UART/UART receive  mask(UART receive){channel=UART2: Con. PD-8 & Con. PD-9 (PD5 & PD6), useStatusOut=off, tsamp=-1}
      mask prompts: useStatusOut "Use status outport"; tsamp "Sample time"
      mask help:
      | Function
      | ==========
      | Reads a byte from the UART reception buffer.
      |
      | Parameters per channel
      | ======================
      | - Select channel
      | - Select if the status output should be enabled.
      |
      | Outputs
      | =======
      | - The value of the receive byte.
      | - When the status output is 0, the reception buffer was empty.
      mask init:
      | uartChannelInfoStr = sfcn_uart_receive_mcb(2, channel, useStatusOut);
      settings: MoveFcn=drawLogos
      mask Help: web('sfcn_uart_receive.html')
      mask TypeOptions channel: UART1: Con. 3-D1 & Con. 3-D0 (PB6 & PB7) | UART2: Con. PD-8 & Con. PD-9 (PD5 & PD6) | UART3: Con. PD-11 & Con. PD-12 (PD8 & PD9) | UART6: Con. UEXT-3 & Con. UEXT-4 (PC6 & PC7)
      mask Display: fprintf('UART receive\n%s', uartChannelInfoStr);patch([240 246 246],[8 14 2],[1 0 0]);patch([248 248 254],[14 2 8],[0 0 0.35]);
  Out1 : Outport
  wires:
  UART receive/1(Out1) -> Out1/1

== system Charge_2_V1/HANcoder STM32 Target - E407-STM32 algorithm/Energy Meter1/Energy_Meter_Recieve/Fequency/Read_Gyro8 ==
  Trigger : TriggerPort  VariantControl=Variant
  UART receive : Subsystem  AncestorBlock=HANcoder_STM32_Target/STM32-E407/UART/UART receive  mask(UART receive){channel=UART2: Con. PD-8 & Con. PD-9 (PD5 & PD6), useStatusOut=off, tsamp=-1}
      mask prompts: useStatusOut "Use status outport"; tsamp "Sample time"
      mask help:
      | Function
      | ==========
      | Reads a byte from the UART reception buffer.
      |
      | Parameters per channel
      | ======================
      | - Select channel
      | - Select if the status output should be enabled.
      |
      | Outputs
      | =======
      | - The value of the receive byte.
      | - When the status output is 0, the reception buffer was empty.
      mask init:
      | uartChannelInfoStr = sfcn_uart_receive_mcb(2, channel, useStatusOut);
      settings: MoveFcn=drawLogos
      mask Help: web('sfcn_uart_receive.html')
      mask TypeOptions channel: UART1: Con. 3-D1 & Con. 3-D0 (PB6 & PB7) | UART2: Con. PD-8 & Con. PD-9 (PD5 & PD6) | UART3: Con. PD-11 & Con. PD-12 (PD8 & PD9) | UART6: Con. UEXT-3 & Con. UEXT-4 (PC6 & PC7)
      mask Display: fprintf('UART receive\n%s', uartChannelInfoStr);patch([240 246 246],[8 14 2],[1 0 0]);patch([248 248 254],[14 2 8],[0 0 0.35]);
  Out1 : Outport
  wires:
  UART receive/1(Out1) -> Out1/1

== system Charge_2_V1/HANcoder STM32 Target - E407-STM32 algorithm/Energy Meter1/Energy_Meter_Recieve/Fequency/Read_Gyro9 ==
  Trigger : TriggerPort  VariantControl=Variant
  UART receive : Subsystem  AncestorBlock=HANcoder_STM32_Target/STM32-E407/UART/UART receive  mask(UART receive){channel=UART2: Con. PD-8 & Con. PD-9 (PD5 & PD6), useStatusOut=off, tsamp=-1}
      mask prompts: useStatusOut "Use status outport"; tsamp "Sample time"
      mask help:
      | Function
      | ==========
      | Reads a byte from the UART reception buffer.
      |
      | Parameters per channel
      | ======================
      | - Select channel
      | - Select if the status output should be enabled.
      |
      | Outputs
      | =======
      | - The value of the receive byte.
      | - When the status output is 0, the reception buffer was empty.
      mask init:
      | uartChannelInfoStr = sfcn_uart_receive_mcb(2, channel, useStatusOut);
      settings: MoveFcn=drawLogos
      mask Help: web('sfcn_uart_receive.html')
      mask TypeOptions channel: UART1: Con. 3-D1 & Con. 3-D0 (PB6 & PB7) | UART2: Con. PD-8 & Con. PD-9 (PD5 & PD6) | UART3: Con. PD-11 & Con. PD-12 (PD8 & PD9) | UART6: Con. UEXT-3 & Con. UEXT-4 (PC6 & PC7)
      mask Display: fprintf('UART receive\n%s', uartChannelInfoStr);patch([240 246 246],[8 14 2],[1 0 0]);patch([248 248 254],[14 2 8],[0 0 0.35]);
  Out1 : Outport
  wires:
  UART receive/1(Out1) -> Out1/1

== system Charge_2_V1/HANcoder STM32 Target - E407-STM32 algorithm/Energy Meter1/Energy_Meter_Recieve/Subsystem/FloatConv1 ==
  In1 : Inport
  In2 : Inport  Port=2
  In3 : Inport  Port=3
  In4 : Inport  Port=4
  Bitwise Operator : simulink/Logic and Bit Operations/Bitwise Operator  logicop=AND  UseBitMask=on  BitMask=bin2dec('01111111')  BitMaskRealWorld=Stored Integer
  Constant : Constant  Value=127  SampleTime=0.1
  Constant1 : Constant  Value=2  SampleTime=0.1
  Constant3 : Constant  Value=8388607  SampleTime=0.1
  Data Type Conversion : DataTypeConversion
  Data Type Conversion1 : DataTypeConversion  OutDataTypeStr=uint32
  Data Type Conversion8 : DataTypeConversion  OutDataTypeStr=uint32
  Gain1 : Gain  Gain=65536
  Gain2 : Gain  Gain=256
  Gain7 : Gain  Gain=1/8388607
  Math Function1 : Math  Operator=pow  SaturateOnIntegerOverflow=on
  Product : Product  OutDataTypeStr=single
  Shift Arithmetic : ArithShift  BitShiftNumber=1  BitShiftDirection=Left
  Shift Arithmetic1 : ArithShift  BitShiftNumber=7  BitShiftDirection=Right
  Sum : Sum  Inputs=|++
  Sum2 : Sum  Inputs=|+-
  Sum3 : Sum  Inputs=++++
  byte5 : Outport  SampleTime=0.1
  wires:
  Math Function1/1 -> Product/1
  Product/1 -> byte5/1
  Gain7/1 -> Product/2
  Constant1/1 -> Math Function1/1
  Sum2/1 -> Math Function1/2
  Constant/1 -> Sum2/2
  Data Type Conversion/1 -> Sum2/1
  Sum/1 -> Data Type Conversion/1
  Shift Arithmetic1/1 -> Sum/2
  Shift Arithmetic/1 -> Sum/1
  In2/1 -> Shift Arithmetic1/1, Bitwise Operator/1
  In1/1 -> Shift Arithmetic/1
  In4/1 -> Sum3/3
  Constant3/1 -> Sum3/4
  Sum3/1 -> Gain7/1
  Bitwise Operator/1 -> Data Type Conversion8/1
  In3/1 -> Data Type Conversion1/1
  Data Type Conversion1/1 -> Gain2/1
  Gain2/1 -> Sum3/2
  Gain1/1 -> Sum3/1
  Data Type Conversion8/1 -> Gain1/1

== system Charge_2_V1/HANcoder STM32 Target - E407-STM32 algorithm/Energy Meter1/Energy_Meter_Recieve/Subsystem/FloatConv2 ==
  In1 : Inport
  In2 : Inport  Port=2
  In3 : Inport  Port=3
  In4 : Inport  Port=4
  Bitwise Operator : simulink/Logic and Bit Operations/Bitwise Operator  logicop=AND  UseBitMask=on  BitMask=bin2dec('01111111')  BitMaskRealWorld=Stored Integer
  Constant : Constant  Value=127  SampleTime=0.1
  Constant1 : Constant  Value=2  SampleTime=0.1
  Constant3 : Constant  Value=8388607  SampleTime=0.1
  Data Type Conversion : DataTypeConversion
  Data Type Conversion1 : DataTypeConversion  OutDataTypeStr=uint32
  Data Type Conversion8 : DataTypeConversion  OutDataTypeStr=uint32
  Gain1 : Gain  Gain=65536
  Gain2 : Gain  Gain=256
  Gain7 : Gain  Gain=1/8388607
  Math Function1 : Math  Operator=pow  SaturateOnIntegerOverflow=on
  Product : Product  OutDataTypeStr=single
  Shift Arithmetic : ArithShift  BitShiftNumber=1  BitShiftDirection=Left
  Shift Arithmetic1 : ArithShift  BitShiftNumber=7  BitShiftDirection=Right
  Sum : Sum  Inputs=|++
  Sum2 : Sum  Inputs=|+-
  Sum3 : Sum  Inputs=++++
  byte5 : Outport  SampleTime=0.1
  wires:
  Data Type Conversion8/1 -> Gain1/1
  Gain1/1 -> Sum3/1
  Gain2/1 -> Sum3/2
  Data Type Conversion1/1 -> Gain2/1
  In3/1 -> Data Type Conversion1/1
  Bitwise Operator/1 -> Data Type Conversion8/1
  Sum3/1 -> Gain7/1
  Constant3/1 -> Sum3/4
  In4/1 -> Sum3/3
  In1/1 -> Shift Arithmetic/1
  In2/1 -> Bitwise Operator/1, Shift Arithmetic1/1
  Shift Arithmetic/1 -> Sum/1
  Shift Arithmetic1/1 -> Sum/2
  Sum/1 -> Data Type Conversion/1
  Data Type Conversion/1 -> Sum2/1
  Constant/1 -> Sum2/2
  Sum2/1 -> Math Function1/2
  Constant1/1 -> Math Function1/1
  Gain7/1 -> Product/2
  Product/1 -> byte5/1
  Math Function1/1 -> Product/1

== system Charge_2_V1/HANcoder STM32 Target - E407-STM32 algorithm/Energy Meter1/Energy_Meter_Recieve/Subsystem/FloatConv3 ==
  In1 : Inport
  In2 : Inport  Port=2
  In3 : Inport  Port=3
  In4 : Inport  Port=4
  Bitwise Operator : simulink/Logic and Bit Operations/Bitwise Operator  logicop=AND  UseBitMask=on  BitMask=bin2dec('01111111')  BitMaskRealWorld=Stored Integer
  Constant : Constant  Value=127  SampleTime=0.1
  Constant1 : Constant  Value=2  SampleTime=0.1
  Constant3 : Constant  Value=8388607  SampleTime=0.1
  Data Type Conversion : DataTypeConversion
  Data Type Conversion1 : DataTypeConversion  OutDataTypeStr=uint32
  Data Type Conversion8 : DataTypeConversion  OutDataTypeStr=uint32
  Gain1 : Gain  Gain=65536
  Gain2 : Gain  Gain=256
  Gain7 : Gain  Gain=1/8388607
  Math Function1 : Math  Operator=pow  SaturateOnIntegerOverflow=on
  Product : Product  OutDataTypeStr=single
  Shift Arithmetic : ArithShift  BitShiftNumber=1  BitShiftDirection=Left
  Shift Arithmetic1 : ArithShift  BitShiftNumber=7  BitShiftDirection=Right
  Sum : Sum  Inputs=|++
  Sum2 : Sum  Inputs=|+-
  Sum3 : Sum  Inputs=++++
  byte5 : Outport  SampleTime=0.1
  wires:
  Math Function1/1 -> Product/1
  Product/1 -> byte5/1
  Gain7/1 -> Product/2
  Constant1/1 -> Math Function1/1
  Sum2/1 -> Math Function1/2
  Constant/1 -> Sum2/2
  Data Type Conversion/1 -> Sum2/1
  Sum/1 -> Data Type Conversion/1
  Shift Arithmetic1/1 -> Sum/2
  Shift Arithmetic/1 -> Sum/1
  In2/1 -> Shift Arithmetic1/1, Bitwise Operator/1
  In1/1 -> Shift Arithmetic/1
  In4/1 -> Sum3/3
  Constant3/1 -> Sum3/4
  Sum3/1 -> Gain7/1
  Bitwise Operator/1 -> Data Type Conversion8/1
  In3/1 -> Data Type Conversion1/1
  Data Type Conversion1/1 -> Gain2/1
  Gain2/1 -> Sum3/2
  Gain1/1 -> Sum3/1
  Data Type Conversion8/1 -> Gain1/1

== system Charge_2_V1/HANcoder STM32 Target - E407-STM32 algorithm/Energy Meter1/Energy_Meter_Recieve/Subsystem/FloatConv4 ==
  In1 : Inport
  In2 : Inport  Port=2
  In3 : Inport  Port=3
  In4 : Inport  Port=4
  Bitwise Operator : simulink/Logic and Bit Operations/Bitwise Operator  logicop=AND  UseBitMask=on  BitMask=bin2dec('01111111')  BitMaskRealWorld=Stored Integer
  Constant : Constant  Value=127  SampleTime=0.1
  Constant1 : Constant  Value=2  SampleTime=0.1
  Constant3 : Constant  Value=8388607  SampleTime=0.1
  Data Type Conversion : DataTypeConversion
  Data Type Conversion1 : DataTypeConversion  OutDataTypeStr=uint32
  Data Type Conversion8 : DataTypeConversion  OutDataTypeStr=uint32
  Gain1 : Gain  Gain=65536
  Gain2 : Gain  Gain=256
  Gain7 : Gain  Gain=1/8388607
  Math Function1 : Math  Operator=pow  SaturateOnIntegerOverflow=on
  Product : Product  OutDataTypeStr=single
  Shift Arithmetic : ArithShift  BitShiftNumber=1  BitShiftDirection=Left
  Shift Arithmetic1 : ArithShift  BitShiftNumber=7  BitShiftDirection=Right
  Sum : Sum  Inputs=|++
  Sum2 : Sum  Inputs=|+-
  Sum3 : Sum  Inputs=++++
  byte5 : Outport  SampleTime=0.1
  wires:
  Data Type Conversion8/1 -> Gain1/1
  Gain1/1 -> Sum3/1
  Gain2/1 -> Sum3/2
  Data Type Conversion1/1 -> Gain2/1
  In3/1 -> Data Type Conversion1/1
  Bitwise Operator/1 -> Data Type Conversion8/1
  Sum3/1 -> Gain7/1
  Constant3/1 -> Sum3/4
  In4/1 -> Sum3/3
  In1/1 -> Shift Arithmetic/1
  In2/1 -> Bitwise Operator/1, Shift Arithmetic1/1
  Shift Arithmetic/1 -> Sum/1
  Shift Arithmetic1/1 -> Sum/2
  Sum/1 -> Data Type Conversion/1
  Data Type Conversion/1 -> Sum2/1
  Constant/1 -> Sum2/2
  Sum2/1 -> Math Function1/2
  Constant1/1 -> Math Function1/1
  Gain7/1 -> Product/2
  Product/1 -> byte5/1
  Math Function1/1 -> Product/1

== system Charge_2_V1/HANcoder STM32 Target - E407-STM32 algorithm/Energy Meter1/Energy_Meter_Recieve/Subsystem/FloatConv5 ==
  In1 : Inport
  In2 : Inport  Port=2
  In3 : Inport  Port=3
  In4 : Inport  Port=4
  Bitwise Operator : simulink/Logic and Bit Operations/Bitwise Operator  logicop=AND  UseBitMask=on  BitMask=bin2dec('01111111')  BitMaskRealWorld=Stored Integer
  Constant : Constant  Value=127  SampleTime=0.1
  Constant1 : Constant  Value=2  SampleTime=0.1
  Constant3 : Constant  Value=8388607  SampleTime=0.1
  Data Type Conversion : DataTypeConversion
  Data Type Conversion1 : DataTypeConversion  OutDataTypeStr=uint32
  Data Type Conversion8 : DataTypeConversion  OutDataTypeStr=uint32
  Gain1 : Gain  Gain=65536
  Gain2 : Gain  Gain=256
  Gain7 : Gain  Gain=1/8388607
  Math Function1 : Math  Operator=pow  SaturateOnIntegerOverflow=on
  Product : Product  OutDataTypeStr=single
  Shift Arithmetic : ArithShift  BitShiftNumber=1  BitShiftDirection=Left
  Shift Arithmetic1 : ArithShift  BitShiftNumber=7  BitShiftDirection=Right
  Sum : Sum  Inputs=|++
  Sum2 : Sum  Inputs=|+-
  Sum3 : Sum  Inputs=++++
  byte5 : Outport  SampleTime=0.1
  wires:
  Math Function1/1 -> Product/1
  Product/1 -> byte5/1
  Gain7/1 -> Product/2
  Constant1/1 -> Math Function1/1
  Sum2/1 -> Math Function1/2
  Constant/1 -> Sum2/2
  Data Type Conversion/1 -> Sum2/1
  Sum/1 -> Data Type Conversion/1
  Shift Arithmetic1/1 -> Sum/2
  Shift Arithmetic/1 -> Sum/1
  In2/1 -> Shift Arithmetic1/1, Bitwise Operator/1
  In1/1 -> Shift Arithmetic/1
  In4/1 -> Sum3/3
  Constant3/1 -> Sum3/4
  Sum3/1 -> Gain7/1
  Bitwise Operator/1 -> Data Type Conversion8/1
  In3/1 -> Data Type Conversion1/1
  Data Type Conversion1/1 -> Gain2/1
  Gain2/1 -> Sum3/2
  Gain1/1 -> Sum3/1
  Data Type Conversion8/1 -> Gain1/1

== system Charge_2_V1/HANcoder STM32 Target - E407-STM32 algorithm/Energy Meter1/Energy_Meter_Recieve/Subsystem/FloatConv6 ==
  In1 : Inport
  In2 : Inport  Port=2
  In3 : Inport  Port=3
  In4 : Inport  Port=4
  Bitwise Operator : simulink/Logic and Bit Operations/Bitwise Operator  logicop=AND  UseBitMask=on  BitMask=bin2dec('01111111')  BitMaskRealWorld=Stored Integer
  Constant : Constant  Value=127  SampleTime=0.1
  Constant1 : Constant  Value=2  SampleTime=0.1
  Constant3 : Constant  Value=8388607  SampleTime=0.1
  Data Type Conversion : DataTypeConversion
  Data Type Conversion1 : DataTypeConversion  OutDataTypeStr=uint32
  Data Type Conversion8 : DataTypeConversion  OutDataTypeStr=uint32
  Gain1 : Gain  Gain=65536
  Gain2 : Gain  Gain=256
  Gain7 : Gain  Gain=1/8388607
  Math Function1 : Math  Operator=pow  SaturateOnIntegerOverflow=on
  Product : Product  OutDataTypeStr=single
  Shift Arithmetic : ArithShift  BitShiftNumber=1  BitShiftDirection=Left
  Shift Arithmetic1 : ArithShift  BitShiftNumber=7  BitShiftDirection=Right
  Sum : Sum  Inputs=|++
  Sum2 : Sum  Inputs=|+-
  Sum3 : Sum  Inputs=++++
  byte5 : Outport  SampleTime=0.1
  wires:
  Data Type Conversion8/1 -> Gain1/1
  Gain1/1 -> Sum3/1
  Gain2/1 -> Sum3/2
  Data Type Conversion1/1 -> Gain2/1
  In3/1 -> Data Type Conversion1/1
  Bitwise Operator/1 -> Data Type Conversion8/1
  Sum3/1 -> Gain7/1
  Constant3/1 -> Sum3/4
  In4/1 -> Sum3/3
  In1/1 -> Shift Arithmetic/1
  In2/1 -> Bitwise Operator/1, Shift Arithmetic1/1
  Shift Arithmetic/1 -> Sum/1
  Shift Arithmetic1/1 -> Sum/2
  Sum/1 -> Data Type Conversion/1
  Data Type Conversion/1 -> Sum2/1
  Constant/1 -> Sum2/2
  Sum2/1 -> Math Function1/2
  Constant1/1 -> Math Function1/1
  Gain7/1 -> Product/2
  Product/1 -> byte5/1
  Math Function1/1 -> Product/1

== system Charge_2_V1/HANcoder STM32 Target - E407-STM32 algorithm/Energy Meter1/Energy_Meter_Recieve/Subsystem/FloatConv7 ==
  In1 : Inport
  In2 : Inport  Port=2
  In3 : Inport  Port=3
  In4 : Inport  Port=4
  Bitwise Operator : simulink/Logic and Bit Operations/Bitwise Operator  logicop=AND  UseBitMask=on  BitMask=bin2dec('01111111')  BitMaskRealWorld=Stored Integer
  Constant : Constant  Value=127  SampleTime=0.1
  Constant1 : Constant  Value=2  SampleTime=0.1
  Constant3 : Constant  Value=8388607  SampleTime=0.1
  Data Type Conversion : DataTypeConversion
  Data Type Conversion1 : DataTypeConversion  OutDataTypeStr=uint32
  Data Type Conversion8 : DataTypeConversion  OutDataTypeStr=uint32
  Gain1 : Gain  Gain=65536
  Gain2 : Gain  Gain=256
  Gain7 : Gain  Gain=1/8388607
  Math Function1 : Math  Operator=pow  SaturateOnIntegerOverflow=on
  Product : Product  OutDataTypeStr=single
  Shift Arithmetic : ArithShift  BitShiftNumber=1  BitShiftDirection=Left
  Shift Arithmetic1 : ArithShift  BitShiftNumber=7  BitShiftDirection=Right
  Sum : Sum  Inputs=|++
  Sum2 : Sum  Inputs=|+-
  Sum3 : Sum  Inputs=++++
  byte5 : Outport  SampleTime=0.1
  wires:
  Math Function1/1 -> Product/1
  Product/1 -> byte5/1
  Gain7/1 -> Product/2
  Constant1/1 -> Math Function1/1
  Sum2/1 -> Math Function1/2
  Constant/1 -> Sum2/2
  Data Type Conversion/1 -> Sum2/1
  Sum/1 -> Data Type Conversion/1
  Shift Arithmetic1/1 -> Sum/2
  Shift Arithmetic/1 -> Sum/1
  In2/1 -> Shift Arithmetic1/1, Bitwise Operator/1
  In1/1 -> Shift Arithmetic/1
  In4/1 -> Sum3/3
  Constant3/1 -> Sum3/4
  Sum3/1 -> Gain7/1
  Bitwise Operator/1 -> Data Type Conversion8/1
  In3/1 -> Data Type Conversion1/1
  Data Type Conversion1/1 -> Gain2/1
  Gain2/1 -> Sum3/2
  Gain1/1 -> Sum3/1
  Data Type Conversion8/1 -> Gain1/1

== system Charge_2_V1/HANcoder STM32 Target - E407-STM32 algorithm/Energy Meter1/Energy_Meter_Recieve/Subsystem1/Power_Meter ==
  note: Write Description for messeages sequences
  In1 : Inport
  In2 : Inport  Port=2
  In3 : Inport  Port=3
  In4 : Inport  Port=4
  In5 : Inport  Port=5
  In6 : Inport  Port=6
  In7 : Inport  Port=7
  In8 : Inport  Port=8
  In9 : Inport  Port=9
  In10 : Inport  Port=10
  In11 : Inport  Port=11
  In12 : Inport  Port=12
  In13 : Inport  Port=13
  " " : simulink/Logic and Bit Operations/Compare To Constant  relop===  const=800  OutDataTypeStr=boolean
  Compare To Constant14 : simulink/Logic and Bit Operations/Compare To Constant  relop===  const=814  OutDataTypeStr=boolean
  Compare To Constant5 : simulink/Logic and Bit Operations/Compare To Constant  relop===  const=801  OutDataTypeStr=boolean
  Current_Phase1 : Subsystem
  Current_phase2 : Subsystem
  Last byte : Subsystem  TreatAsAtomicUnit=on
  Read_Gyro11 : Subsystem  TreatAsAtomicUnit=on
  Read_Gyro6 : Subsystem  TreatAsAtomicUnit=on
  Subsystem : Subsystem
  wires:
  " "/1 -> Read_Gyro11/Trigger
  In1/1 -> Current_Phase1/1(In1), Current_phase2/1(In1), Subsystem/1(In1), Compare To Constant14/1, Compare To Constant5/1, " "/1
  Compare To Constant5/1 -> Read_Gyro6/Trigger
  Compare To Constant14/1 -> Last byte/Trigger
  In2/1 -> Current_Phase1/2(In2)
  In3/1 -> Current_Phase1/3(In3)
  In4/1 -> Current_Phase1/4(In4)
  In5/1 -> Current_Phase1/5(In5)
  In6/1 -> Current_phase2/2(In6)
  In7/1 -> Current_phase2/3(In7)
  In8/1 -> Current_phase2/4(In8)
  In9/1 -> Current_phase2/5(In9)
  In10/1 -> Subsystem/2(In10)
  In11/1 -> Subsystem/3(In11)
  In12/1 -> Subsystem/4(In12)
  In13/1 -> Subsystem/5(In13)
